simulink model "larix2"  (R2020b)
settings: Solver=FixedStepDiscrete  StartTime=0.0  StopTime=inf  FixedStep=0.002  RelTol=1e-3
PostLoadFcn:
  | load('ThrustTable.mat');
InitFcn:
  | run init.m
  | init()
values from neighbouring files (symbols this model uses):
  blimp = inertias()    [init.m]
  eul_0 = [-45*pi/180 0 0]    [init.m]
  g = 9.810    (= 9.81)    [init.m]
libraries: slpidlib x10, simulink x10, sharedtransform x1
settings Model: Creator=ac114611  LastModifiedBy=wendelin
settings DataIOCC: ReturnWorkspaceOutputs=off
settings OptimizationCC: BlockReduction=off  DefaultParameterBehavior=Inlined  BufferReuse=off  EnhancedBackFolding=on  PassReuseOutputArgsAs=Individual arguments  MaxStackSize=64  OptimizeBlockOrder=speed  DifferentSizesBufferReuse=on  EfficientTunableParamExpr=on
settings DebuggingCC: ParameterPrecisionLossMsg=none  ParameterTunabilityLossMsg=error  ArithmeticOperatorsInVariantConditions=warning
settings HardwareCC: ProdBitPerPointer=32  ProdBitPerSizeT=32  ProdBitPerPtrDiffT=32  ProdLargestAtomicInteger=Long  ProdLargestAtomicFloat=Double  ProdWordSize=32  ProdHWDeviceType=ARM Compatible->ARM Cortex  TargetBitPerLong=64  TargetBitPerPointer=64  TargetBitPerSizeT=64  TargetBitPerPtrDiffT=64  TargetLongLongMode=on  TargetIntDivRoundTo=Zero  TargetEndianess=LittleEndian  TargetWordSize=64  TargetHWDeviceType=MATLAB Host  ProdEqTarget=off
settings SFSimCC: SimUseLocalCustomCode=off  MATLABDynamicMemAlloc=off  CustomCodeUndefinedFunction=UseInterfaceOnly
settings RTWCC: Description=Embedded Coder  SystemTargetFile=ert.tlc  GenCodeOnly=on  PackageName=larix2_codegen.zip  TemplateMakefile=ert_default_tmf  RTWUseLocalCustomCode=off  Toolchain=GNU gcc/g++ | gmake (64-bit Linux)  IncludeHyperlinkInReport=on  GenerateCodeMetricsReport=on
settings CodeAppCC: ForceParamTrailComments=on  IgnoreCustomStorageClasses=off  OperatorAnnotations=on  SimulinkDataObjDesc=on  SFDataObjDesc=on  InsertBlockDesc=on
settings ERTTargetCC: TargetLangStandard=C99 (ISO)  SupportVariableSizeSignals=on  InlinedParameterPlacement=NonHierarchical  ERTCustomFileTemplate=example_file_process.tlc

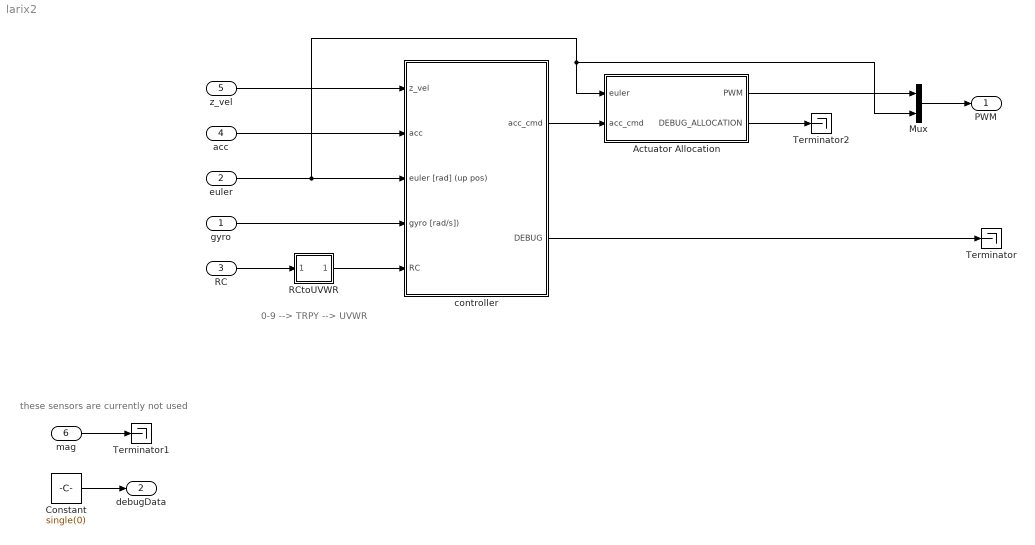
== system larix2 ==
  note: 0-9 --> TRPY --> UVWR
  note: these sensors are currently not used
  gyro : Inport  OutDataTypeStr=single  PortDimensions=3
  euler : Inport  Port=2  OutDataTypeStr=single  PortDimensions=3
  RC : Inport  Port=3  OutDataTypeStr=single  PortDimensions=10
  acc : Inport  Port=4  OutDataTypeStr=single  PortDimensions=3
  "z_vel " : Inport  Port=5  OutDataTypeStr=single  PortDimensions=1
  mag : Inport  Port=6  OutDataTypeStr=single  PortDimensions=3
  Actuator Allocation : Subsystem
  Constant : Constant  Value=single(0)
  Mux : Mux  Inputs=2
  RCtoUVWR : Subsystem
  Terminator : Terminator
  Terminator1 : Terminator
  Terminator2 : Terminator
  controller : Subsystem
  PWM : Outport  OutDataTypeStr=single  VectorParamsAs1DForOutWhenUnconnected=off
  debugData : Outport  Port=2
  wires:
  mag/1 -> Terminator1/1
  Actuator Allocation/1(PWM) -> Mux/1
  "z_vel "/1 -> controller/1(z_vel)
  acc/1 -> controller/2(acc)
  euler/1 -> Mux/2, Actuator Allocation/1(euler), controller/3(euler [rad] (up pos))
  gyro/1 -> controller/4(gyro [rad/s]))
  Constant/1 -> debugData/1
  Mux/1 -> PWM/1
  controller/2(DEBUG) -> Terminator/1
  controller/1(acc_cmd) -> Actuator Allocation/2(acc_cmd)
  RC/1 -> RCtoUVWR/1(RC)
  RCtoUVWR/1(Out1) -> controller/5(RC)
  Actuator Allocation/2(DEBUG_ALLOCATION) -> Terminator2/1

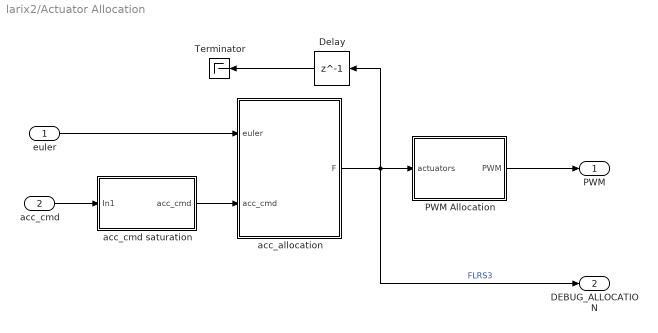
== system larix2/Actuator Allocation ==
  euler : Inport
  acc_cmd : Inport  Port=2
  Delay : Delay  DelayLength=1
  PWM Allocation : Subsystem
  Terminator : Terminator
  acc_allocation : MATLAB Function  TreatAsAtomicUnit=on
  acc_cmd saturation : Subsystem
  PWM : Outport
  DEBUG_ALLOCATION : Outport  Port=2
  wires:
  acc_cmd/1 -> acc_cmd saturation/1(In1)
  acc_cmd saturation/1(acc_cmd) -> acc_allocation/2(acc_cmd)
  euler/1 -> acc_allocation/1(euler)
  PWM Allocation/1(PWM) -> PWM/1
  acc_allocation/1(F) -> DEBUG_ALLOCATION/1, PWM Allocation/1(actuators), Delay/1  "FLRS3"
  Delay/1 -> Terminator/1

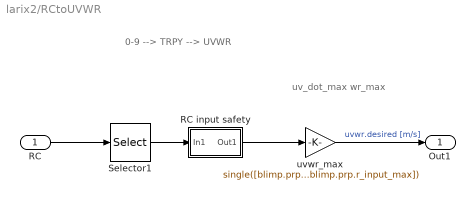
== system larix2/RCtoUVWR ==
  note: uv_dot_max
      | wr_max
  note: 0-9 --> TRPY --> UVWR
  RC : Inport  PortDimensions=10
  RC input safety : Subsystem
  Selector1 : Selector  IndexMode=Zero-based  InputPortWidth=10  IndexOptions=Index vector (dialog)  Indices=[2 1 0 3]  OutputSizes=1
  uvwr_max : Gain  Gain=single([blimp.prp.du_input_max, blimp.prp.dv_input_max, blimp.prp.w_input_max, blimp.prp.r_input_max])
  Out1 : Outport
  wires:
  RC/1 -> Selector1/1
  RC input safety/1(Out1) -> uvwr_max/1
  Selector1/1 -> RC input safety/1(In1)
  uvwr_max/1 -> Out1/1  "uvwr.desired [m/s]"

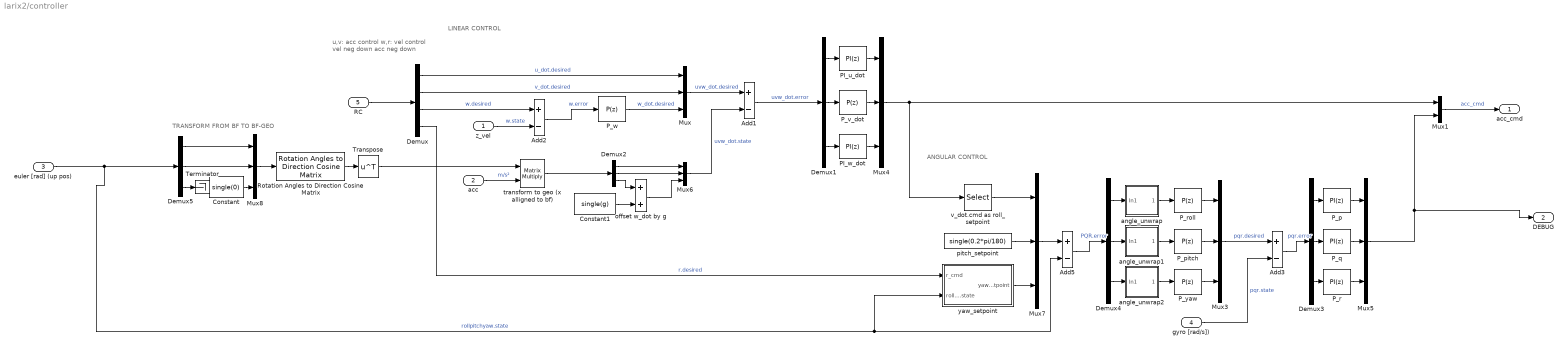
== system larix2/controller ==
  note: TRANSFORM FROM BF TO BF-GEO
  note: u,v: acc control
      | w,r: vel control
      |
      | vel neg down
      | acc neg down
  note: LINEAR CONTROL
  note: ANGULAR CONTROL
  z_vel : Inport  PortDimensions=1
  acc : Inport  Port=2  PortDimensions=3
  euler [rad] (up pos) : Inport  Port=3  PortDimensions=3
  gyro [rad/s]) : Inport  Port=4  PortDimensions=3
  RC : Inport  Port=5
  Add{1..3,5} (4 alike) : Sum  Inputs=+-
  Constant : Constant  Value=single(0)
  Constant1 : Constant  Value=single(g)
  Demux : Demux
  Demux{1..5} (5 alike) : Demux  Outputs=3
  Mux{,3..8} (7 alike) : Mux  Inputs=3
  Mux1 : Mux  Inputs=2
  PI_u_dot : slpidlib/PID Controller  Controller=PI  Form=Parallel  TimeDomain=Discrete-time  UseExternalTs=off  SampleTime=-1  IntegratorMethod=Trapezoidal  FilterMethod=Forward Euler  ControllerParametersSource=internal  P=0.15  I=0.05  D=0  UseFilter=on  N=100  TunerSelectOption=Transfer Function Based (PID Tuner App)  InitialConditionSource=internal  InitialConditionForIntegrator=0  InitialConditionForFilter=0  DifferentiatorICPrevScaledInput=0  ExternalReset=none  TrackingMode=off  Kt=1  LimitOutput=off  SatLimitsSource=internal  UpperSaturationLimit=0.4*g  LowerSaturationLimit=-0.4*g  LinearizeAsGain=off  AntiWindupMode=none  Kb=1  POutMin=[]  POutMax=[]  IOutMin=[]  IOutMax=[]  DOutMin=[]  DOutMax=[]  NOutMin=[]  NOutMax=[]  SumOutMin=[]  SumOutMax=[]  SaturationOutMin=[]  SaturationOutMax=[]  PParamMin=[]  PParamMax=[]  IParamMin=[]  IParamMax=[]  DParamMin=[]  DParamMax=[]  NParamMin=[]  NParamMax=[]  KbParamMin=[]  KbParamMax=[]  KtParamMin=[]  KtParamMax=[]  KbOutMin=[]  KbOutMax=[]  KtOutMin=[]  KtOutMax=[]  IntegratorOutMin=[]  IntegratorOutMax=[]  FilterOutMin=[]  FilterOutMax=[]  SumI1OutMin=[]  SumI1OutMax=[]  SumI2OutMin=[]  SumI2OutMax=[]  SumI3OutMin=[]  SumI3OutMax=[]  SumI4OutMin=[]  SumI4OutMax=[]  SumDOutMin=[]  SumDOutMax=[]  DifferentiatorOutMin=[]  DifferentiatorOutMax=[]  FilterDiffOutCoefMin=[]  FilterDiffOutCoefMax=[]  ReciprocalOutMin=[]  ReciprocalOutMax=[]  SumDenOutMin=[]  SumDenOutMax=[]  SumNumOutMin=[]  SumNumOutMax=[]  DivideOutMin=[]  DivideOutMax=[]  UdiffTsProdOutMin=[]  UdiffTsProdOutMax=[]  NTsProdOutMin=[]  NTsProdOutMax=[]  UintegralTsProdOutMin=[]  UintegralTsProdOutMax=[]  UngainTsProdOutMin=[]  UngainTsProdOutMax=[]  IntegratorContinuousStateAttributes=''  IntegratorStateMustResolveToSignalObject=off  IntegratorRTWStateStorageClass=Auto  FilterContinuousStateAttributes=''  FilterStateMustResolveToSignalObject=off  FilterRTWStateStorageClass=Auto  ParallelPVariant=InternalParameters  IdealPVariant=Disabled  IVariant=InternalParameters  DVariant=Disabled  IntegratorVariant=Discrete  SatVariant=Disabled  AWVariant=Passthrough  PCopyVariant=Disabled  TRVariant=Disabled  FdbkBlocksVariant=Forward  IdealPFdbkVariant=Disabled  SatFdbkVariant=Disabled  DerivativeFilterVariant=Disabled  NVariant=Disabled  NCopyVariant=Disabled_SignalSpec  FilterICVariant=Disabled  IntegratorICVariant=InternalICs  ExternalResetVariant=Disabled  TRSumVariant=Passthrough  SumFdbkVariant=Disabled  SumVariant=Sum_PI  TsampFilterVariant=InternalTs  TsampNgainVariant=Passthrough  TsampIntegralVariant=Passthrough  ExternalSaturationOutDataTypeStr=Inherit: Same as second input
  PI_w_dot : slpidlib/PID Controller  Controller=PI  Form=Parallel  TimeDomain=Discrete-time  UseExternalTs=off  SampleTime=-1  IntegratorMethod=Forward Euler  FilterMethod=Forward Euler  ControllerParametersSource=internal  P=1.8  I=1.4  D=0  UseFilter=on  N=100  TunerSelectOption=Transfer Function Based (PID Tuner App)  InitialConditionSource=internal  InitialConditionForIntegrator=0  InitialConditionForFilter=0  DifferentiatorICPrevScaledInput=0  ExternalReset=none  TrackingMode=off  Kt=1  LimitOutput=off  SatLimitsSource=internal  UpperSaturationLimit=inf  LowerSaturationLimit=0  LinearizeAsGain=off  AntiWindupMode=none  Kb=1  POutMin=[]  POutMax=[]  IOutMin=[]  IOutMax=[]  DOutMin=[]  DOutMax=[]  NOutMin=[]  NOutMax=[]  SumOutMin=[]  SumOutMax=[]  SaturationOutMin=[]  SaturationOutMax=[]  PParamMin=[]  PParamMax=[]  IParamMin=[]  IParamMax=[]  DParamMin=[]  DParamMax=[]  NParamMin=[]  NParamMax=[]  KbParamMin=[]  KbParamMax=[]  KtParamMin=[]  KtParamMax=[]  KbOutMin=[]  KbOutMax=[]  KtOutMin=[]  KtOutMax=[]  IntegratorOutMin=[]  IntegratorOutMax=[]  FilterOutMin=[]  FilterOutMax=[]  SumI1OutMin=[]  SumI1OutMax=[]  SumI2OutMin=[]  SumI2OutMax=[]  SumI3OutMin=[]  SumI3OutMax=[]  SumI4OutMin=[]  SumI4OutMax=[]  SumDOutMin=[]  SumDOutMax=[]  DifferentiatorOutMin=[]  DifferentiatorOutMax=[]  FilterDiffOutCoefMin=[]  FilterDiffOutCoefMax=[]  ReciprocalOutMin=[]  ReciprocalOutMax=[]  SumDenOutMin=[]  SumDenOutMax=[]  SumNumOutMin=[]  SumNumOutMax=[]  DivideOutMin=[]  DivideOutMax=[]  UdiffTsProdOutMin=[]  UdiffTsProdOutMax=[]  NTsProdOutMin=[]  NTsProdOutMax=[]  UintegralTsProdOutMin=[]  UintegralTsProdOutMax=[]  UngainTsProdOutMin=[]  UngainTsProdOutMax=[]  IntegratorContinuousStateAttributes=''  IntegratorStateMustResolveToSignalObject=off  IntegratorRTWStateStorageClass=Auto  FilterContinuousStateAttributes=''  FilterStateMustResolveToSignalObject=off  FilterRTWStateStorageClass=Auto  ParallelPVariant=InternalParameters  IdealPVariant=Disabled  IVariant=InternalParameters  DVariant=Disabled  IntegratorVariant=Discrete  SatVariant=Disabled  AWVariant=Passthrough  PCopyVariant=Disabled  TRVariant=Disabled  FdbkBlocksVariant=Forward  IdealPFdbkVariant=Disabled  SatFdbkVariant=Disabled  DerivativeFilterVariant=Disabled  NVariant=Disabled  NCopyVariant=Disabled_SignalSpec  FilterICVariant=Disabled  IntegratorICVariant=InternalICs  ExternalResetVariant=Disabled  TRSumVariant=Passthrough  SumFdbkVariant=Disabled  SumVariant=Sum_PI  TsampFilterVariant=InternalTs  TsampNgainVariant=Passthrough  TsampIntegralVariant=Passthrough  ExternalSaturationOutDataTypeStr=Inherit: Same as second input
  P_p : slpidlib/PID Controller  Controller=PI  Form=Parallel  TimeDomain=Discrete-time  UseExternalTs=off  SampleTime=-1  IntegratorMethod=Forward Euler  FilterMethod=Forward Euler  ControllerParametersSource=internal  P=0.4  I=10  D=0  UseFilter=on  N=100  TunerSelectOption=Transfer Function Based (PID Tuner App)  InitialConditionSource=internal  InitialConditionForIntegrator=0  InitialConditionForFilter=0  DifferentiatorICPrevScaledInput=0  ExternalReset=none  TrackingMode=off  Kt=1  LimitOutput=off  SatLimitsSource=internal  UpperSaturationLimit=inf  LowerSaturationLimit=-inf  LinearizeAsGain=on  AntiWindupMode=none  Kb=1  POutMin=[]  POutMax=[]  IOutMin=[]  IOutMax=[]  DOutMin=[]  DOutMax=[]  NOutMin=[]  NOutMax=[]  SumOutMin=[]  SumOutMax=[]  SaturationOutMin=[]  SaturationOutMax=[]  PParamMin=[]  PParamMax=[]  IParamMin=[]  IParamMax=[]  DParamMin=[]  DParamMax=[]  NParamMin=[]  NParamMax=[]  KbParamMin=[]  KbParamMax=[]  KtParamMin=[]  KtParamMax=[]  KbOutMin=[]  KbOutMax=[]  KtOutMin=[]  KtOutMax=[]  IntegratorOutMin=[]  IntegratorOutMax=[]  FilterOutMin=[]  FilterOutMax=[]  SumI1OutMin=[]  SumI1OutMax=[]  SumI2OutMin=[]  SumI2OutMax=[]  SumI3OutMin=[]  SumI3OutMax=[]  SumI4OutMin=[]  SumI4OutMax=[]  SumDOutMin=[]  SumDOutMax=[]  DifferentiatorOutMin=[]  DifferentiatorOutMax=[]  FilterDiffOutCoefMin=[]  FilterDiffOutCoefMax=[]  ReciprocalOutMin=[]  ReciprocalOutMax=[]  SumDenOutMin=[]  SumDenOutMax=[]  SumNumOutMin=[]  SumNumOutMax=[]  DivideOutMin=[]  DivideOutMax=[]  UdiffTsProdOutMin=[]  UdiffTsProdOutMax=[]  NTsProdOutMin=[]  NTsProdOutMax=[]  UintegralTsProdOutMin=[]  UintegralTsProdOutMax=[]  UngainTsProdOutMin=[]  UngainTsProdOutMax=[]  IntegratorContinuousStateAttributes=''  IntegratorStateMustResolveToSignalObject=off  IntegratorRTWStateStorageClass=Auto  FilterContinuousStateAttributes=''  FilterStateMustResolveToSignalObject=off  FilterRTWStateStorageClass=Auto  ParallelPVariant=InternalParameters  IdealPVariant=Disabled  IVariant=InternalParameters  DVariant=Disabled  IntegratorVariant=Discrete  SatVariant=Disabled  AWVariant=Passthrough  PCopyVariant=Disabled  TRVariant=Disabled  FdbkBlocksVariant=Forward  IdealPFdbkVariant=Disabled  SatFdbkVariant=Disabled  DerivativeFilterVariant=Disabled  NVariant=Disabled  NCopyVariant=Disabled_SignalSpec  FilterICVariant=Disabled  IntegratorICVariant=InternalICs  ExternalResetVariant=Disabled  TRSumVariant=Passthrough  SumFdbkVariant=Disabled  SumVariant=Sum_PI  TsampFilterVariant=InternalTs  TsampNgainVariant=Passthrough  TsampIntegralVariant=Passthrough  ExternalSaturationOutDataTypeStr=Inherit: Same as second input
  P_pitch : slpidlib/PID Controller  Controller=P  Form=Parallel  TimeDomain=Discrete-time  UseExternalTs=off  SampleTime=-1  IntegratorMethod=Forward Euler  FilterMethod=Forward Euler  ControllerParametersSource=internal  P=1  I=0  D=0  UseFilter=on  N=100  TunerSelectOption=Transfer Function Based (PID Tuner App)  InitialConditionSource=internal  InitialConditionForIntegrator=0  InitialConditionForFilter=0  DifferentiatorICPrevScaledInput=0  ExternalReset=none  TrackingMode=off  Kt=1  LimitOutput=off  SatLimitsSource=internal  UpperSaturationLimit=inf  LowerSaturationLimit=-inf  LinearizeAsGain=on  AntiWindupMode=none  Kb=1  POutMin=[]  POutMax=[]  IOutMin=[]  IOutMax=[]  DOutMin=[]  DOutMax=[]  NOutMin=[]  NOutMax=[]  SumOutMin=[]  SumOutMax=[]  SaturationOutMin=[]  SaturationOutMax=[]  PParamMin=[]  PParamMax=[]  IParamMin=[]  IParamMax=[]  DParamMin=[]  DParamMax=[]  NParamMin=[]  NParamMax=[]  KbParamMin=[]  KbParamMax=[]  KtParamMin=[]  KtParamMax=[]  KbOutMin=[]  KbOutMax=[]  KtOutMin=[]  KtOutMax=[]  IntegratorOutMin=[]  IntegratorOutMax=[]  FilterOutMin=[]  FilterOutMax=[]  SumI1OutMin=[]  SumI1OutMax=[]  SumI2OutMin=[]  SumI2OutMax=[]  SumI3OutMin=[]  SumI3OutMax=[]  SumI4OutMin=[]  SumI4OutMax=[]  SumDOutMin=[]  SumDOutMax=[]  DifferentiatorOutMin=[]  DifferentiatorOutMax=[]  FilterDiffOutCoefMin=[]  FilterDiffOutCoefMax=[]  ReciprocalOutMin=[]  ReciprocalOutMax=[]  SumDenOutMin=[]  SumDenOutMax=[]  SumNumOutMin=[]  SumNumOutMax=[]  DivideOutMin=[]  DivideOutMax=[]  UdiffTsProdOutMin=[]  UdiffTsProdOutMax=[]  NTsProdOutMin=[]  NTsProdOutMax=[]  UintegralTsProdOutMin=[]  UintegralTsProdOutMax=[]  UngainTsProdOutMin=[]  UngainTsProdOutMax=[]  IntegratorContinuousStateAttributes=''  IntegratorStateMustResolveToSignalObject=off  IntegratorRTWStateStorageClass=Auto  FilterContinuousStateAttributes=''  FilterStateMustResolveToSignalObject=off  FilterRTWStateStorageClass=Auto  ParallelPVariant=InternalParameters  IdealPVariant=Disabled  IVariant=Disabled  DVariant=Disabled  IntegratorVariant=Disabled  SatVariant=Disabled  AWVariant=Disabled  PCopyVariant=Disabled  TRVariant=Disabled  FdbkBlocksVariant=Forward  IdealPFdbkVariant=Disabled  SatFdbkVariant=Disabled  DerivativeFilterVariant=Disabled  NVariant=Disabled  NCopyVariant=Disabled_SignalSpec  FilterICVariant=Disabled  IntegratorICVariant=Disabled  ExternalResetVariant=Disabled  TRSumVariant=Passthrough  SumFdbkVariant=Disabled  SumVariant=Passthrough_P  TsampFilterVariant=InternalTs  TsampNgainVariant=Passthrough  TsampIntegralVariant=Disabled_SignalSpec  ExternalSaturationOutDataTypeStr=Inherit: Same as second input
  P_q : slpidlib/PID Controller  Controller=PI  Form=Parallel  TimeDomain=Discrete-time  UseExternalTs=off  SampleTime=-1  IntegratorMethod=Forward Euler  FilterMethod=Forward Euler  ControllerParametersSource=internal  P=1  I=0  D=0  UseFilter=on  N=100  TunerSelectOption=Transfer Function Based (PID Tuner App)  InitialConditionSource=internal  InitialConditionForIntegrator=0  InitialConditionForFilter=0  DifferentiatorICPrevScaledInput=0  ExternalReset=none  TrackingMode=off  Kt=1  LimitOutput=off  SatLimitsSource=internal  UpperSaturationLimit=inf  LowerSaturationLimit=-inf  LinearizeAsGain=on  AntiWindupMode=none  Kb=1  POutMin=[]  POutMax=[]  IOutMin=[]  IOutMax=[]  DOutMin=[]  DOutMax=[]  NOutMin=[]  NOutMax=[]  SumOutMin=[]  SumOutMax=[]  SaturationOutMin=[]  SaturationOutMax=[]  PParamMin=[]  PParamMax=[]  IParamMin=[]  IParamMax=[]  DParamMin=[]  DParamMax=[]  NParamMin=[]  NParamMax=[]  KbParamMin=[]  KbParamMax=[]  KtParamMin=[]  KtParamMax=[]  KbOutMin=[]  KbOutMax=[]  KtOutMin=[]  KtOutMax=[]  IntegratorOutMin=[]  IntegratorOutMax=[]  FilterOutMin=[]  FilterOutMax=[]  SumI1OutMin=[]  SumI1OutMax=[]  SumI2OutMin=[]  SumI2OutMax=[]  SumI3OutMin=[]  SumI3OutMax=[]  SumI4OutMin=[]  SumI4OutMax=[]  SumDOutMin=[]  SumDOutMax=[]  DifferentiatorOutMin=[]  DifferentiatorOutMax=[]  FilterDiffOutCoefMin=[]  FilterDiffOutCoefMax=[]  ReciprocalOutMin=[]  ReciprocalOutMax=[]  SumDenOutMin=[]  SumDenOutMax=[]  SumNumOutMin=[]  SumNumOutMax=[]  DivideOutMin=[]  DivideOutMax=[]  UdiffTsProdOutMin=[]  UdiffTsProdOutMax=[]  NTsProdOutMin=[]  NTsProdOutMax=[]  UintegralTsProdOutMin=[]  UintegralTsProdOutMax=[]  UngainTsProdOutMin=[]  UngainTsProdOutMax=[]  IntegratorContinuousStateAttributes=''  IntegratorStateMustResolveToSignalObject=off  IntegratorRTWStateStorageClass=Auto  FilterContinuousStateAttributes=''  FilterStateMustResolveToSignalObject=off  FilterRTWStateStorageClass=Auto  ParallelPVariant=InternalParameters  IdealPVariant=Disabled  IVariant=InternalParameters  DVariant=Disabled  IntegratorVariant=Discrete  SatVariant=Disabled  AWVariant=Passthrough  PCopyVariant=Disabled  TRVariant=Disabled  FdbkBlocksVariant=Forward  IdealPFdbkVariant=Disabled  SatFdbkVariant=Disabled  DerivativeFilterVariant=Disabled  NVariant=Disabled  NCopyVariant=Disabled_SignalSpec  FilterICVariant=Disabled  IntegratorICVariant=InternalICs  ExternalResetVariant=Disabled  TRSumVariant=Passthrough  SumFdbkVariant=Disabled  SumVariant=Sum_PI  TsampFilterVariant=InternalTs  TsampNgainVariant=Passthrough  TsampIntegralVariant=Passthrough  ExternalSaturationOutDataTypeStr=Inherit: Same as second input
  P_r : slpidlib/PID Controller  Controller=PI  Form=Parallel  TimeDomain=Discrete-time  UseExternalTs=off  SampleTime=-1  IntegratorMethod=Forward Euler  FilterMethod=Forward Euler  ControllerParametersSource=internal  P=0.5  I=0.2  D=0  UseFilter=on  N=100  TunerSelectOption=Transfer Function Based (PID Tuner App)  InitialConditionSource=internal  InitialConditionForIntegrator=0  InitialConditionForFilter=0  DifferentiatorICPrevScaledInput=0  ExternalReset=none  TrackingMode=off  Kt=1  LimitOutput=off  SatLimitsSource=internal  UpperSaturationLimit=inf  LowerSaturationLimit=-inf  LinearizeAsGain=on  AntiWindupMode=none  Kb=1  POutMin=[]  POutMax=[]  IOutMin=[]  IOutMax=[]  DOutMin=[]  DOutMax=[]  NOutMin=[]  NOutMax=[]  SumOutMin=[]  SumOutMax=[]  SaturationOutMin=[]  SaturationOutMax=[]  PParamMin=[]  PParamMax=[]  IParamMin=[]  IParamMax=[]  DParamMin=[]  DParamMax=[]  NParamMin=[]  NParamMax=[]  KbParamMin=[]  KbParamMax=[]  KtParamMin=[]  KtParamMax=[]  KbOutMin=[]  KbOutMax=[]  KtOutMin=[]  KtOutMax=[]  IntegratorOutMin=[]  IntegratorOutMax=[]  FilterOutMin=[]  FilterOutMax=[]  SumI1OutMin=[]  SumI1OutMax=[]  SumI2OutMin=[]  SumI2OutMax=[]  SumI3OutMin=[]  SumI3OutMax=[]  SumI4OutMin=[]  SumI4OutMax=[]  SumDOutMin=[]  SumDOutMax=[]  DifferentiatorOutMin=[]  DifferentiatorOutMax=[]  FilterDiffOutCoefMin=[]  FilterDiffOutCoefMax=[]  ReciprocalOutMin=[]  ReciprocalOutMax=[]  SumDenOutMin=[]  SumDenOutMax=[]  SumNumOutMin=[]  SumNumOutMax=[]  DivideOutMin=[]  DivideOutMax=[]  UdiffTsProdOutMin=[]  UdiffTsProdOutMax=[]  NTsProdOutMin=[]  NTsProdOutMax=[]  UintegralTsProdOutMin=[]  UintegralTsProdOutMax=[]  UngainTsProdOutMin=[]  UngainTsProdOutMax=[]  IntegratorContinuousStateAttributes=''  IntegratorStateMustResolveToSignalObject=off  IntegratorRTWStateStorageClass=Auto  FilterContinuousStateAttributes=''  FilterStateMustResolveToSignalObject=off  FilterRTWStateStorageClass=Auto  ParallelPVariant=InternalParameters  IdealPVariant=Disabled  IVariant=InternalParameters  DVariant=Disabled  IntegratorVariant=Discrete  SatVariant=Disabled  AWVariant=Passthrough  PCopyVariant=Disabled  TRVariant=Disabled  FdbkBlocksVariant=Forward  IdealPFdbkVariant=Disabled  SatFdbkVariant=Disabled  DerivativeFilterVariant=Disabled  NVariant=Disabled  NCopyVariant=Disabled_SignalSpec  FilterICVariant=Disabled  IntegratorICVariant=InternalICs  ExternalResetVariant=Disabled  TRSumVariant=Passthrough  SumFdbkVariant=Disabled  SumVariant=Sum_PI  TsampFilterVariant=InternalTs  TsampNgainVariant=Passthrough  TsampIntegralVariant=Passthrough  ExternalSaturationOutDataTypeStr=Inherit: Same as second input
  P_roll : slpidlib/PID Controller  Controller=P  Form=Parallel  TimeDomain=Discrete-time  UseExternalTs=off  SampleTime=-1  IntegratorMethod=Forward Euler  FilterMethod=Forward Euler  ControllerParametersSource=internal  P=2  I=0  D=0  UseFilter=on  N=100  TunerSelectOption=Transfer Function Based (PID Tuner App)  InitialConditionSource=internal  InitialConditionForIntegrator=0  InitialConditionForFilter=0  DifferentiatorICPrevScaledInput=0  ExternalReset=none  TrackingMode=off  Kt=1  LimitOutput=off  SatLimitsSource=internal  UpperSaturationLimit=inf  LowerSaturationLimit=-inf  LinearizeAsGain=on  AntiWindupMode=none  Kb=1  POutMin=[]  POutMax=[]  IOutMin=[]  IOutMax=[]  DOutMin=[]  DOutMax=[]  NOutMin=[]  NOutMax=[]  SumOutMin=[]  SumOutMax=[]  SaturationOutMin=[]  SaturationOutMax=[]  PParamMin=[]  PParamMax=[]  IParamMin=[]  IParamMax=[]  DParamMin=[]  DParamMax=[]  NParamMin=[]  NParamMax=[]  KbParamMin=[]  KbParamMax=[]  KtParamMin=[]  KtParamMax=[]  KbOutMin=[]  KbOutMax=[]  KtOutMin=[]  KtOutMax=[]  IntegratorOutMin=[]  IntegratorOutMax=[]  FilterOutMin=[]  FilterOutMax=[]  SumI1OutMin=[]  SumI1OutMax=[]  SumI2OutMin=[]  SumI2OutMax=[]  SumI3OutMin=[]  SumI3OutMax=[]  SumI4OutMin=[]  SumI4OutMax=[]  SumDOutMin=[]  SumDOutMax=[]  DifferentiatorOutMin=[]  DifferentiatorOutMax=[]  FilterDiffOutCoefMin=[]  FilterDiffOutCoefMax=[]  ReciprocalOutMin=[]  ReciprocalOutMax=[]  SumDenOutMin=[]  SumDenOutMax=[]  SumNumOutMin=[]  SumNumOutMax=[]  DivideOutMin=[]  DivideOutMax=[]  UdiffTsProdOutMin=[]  UdiffTsProdOutMax=[]  NTsProdOutMin=[]  NTsProdOutMax=[]  UintegralTsProdOutMin=[]  UintegralTsProdOutMax=[]  UngainTsProdOutMin=[]  UngainTsProdOutMax=[]  IntegratorContinuousStateAttributes=''  IntegratorStateMustResolveToSignalObject=off  IntegratorRTWStateStorageClass=Auto  FilterContinuousStateAttributes=''  FilterStateMustResolveToSignalObject=off  FilterRTWStateStorageClass=Auto  ParallelPVariant=InternalParameters  IdealPVariant=Disabled  IVariant=Disabled  DVariant=Disabled  IntegratorVariant=Disabled  SatVariant=Disabled  AWVariant=Disabled  PCopyVariant=Disabled  TRVariant=Disabled  FdbkBlocksVariant=Forward  IdealPFdbkVariant=Disabled  SatFdbkVariant=Disabled  DerivativeFilterVariant=Disabled  NVariant=Disabled  NCopyVariant=Disabled_SignalSpec  FilterICVariant=Disabled  IntegratorICVariant=Disabled  ExternalResetVariant=Disabled  TRSumVariant=Passthrough  SumFdbkVariant=Disabled  SumVariant=Passthrough_P  TsampFilterVariant=InternalTs  TsampNgainVariant=Passthrough  TsampIntegralVariant=Disabled_SignalSpec  ExternalSaturationOutDataTypeStr=Inherit: Same as second input
  P_v_dot : slpidlib/PID Controller  Controller=P  Form=Parallel  TimeDomain=Discrete-time  UseExternalTs=off  SampleTime=-1  IntegratorMethod=Forward Euler  FilterMethod=Forward Euler  ControllerParametersSource=internal  P=2.5 *pi/180  I=1  D=0  UseFilter=on  N=100  TunerSelectOption=Transfer Function Based (PID Tuner App)  InitialConditionSource=internal  InitialConditionForIntegrator=0  InitialConditionForFilter=0  DifferentiatorICPrevScaledInput=0  ExternalReset=none  TrackingMode=off  Kt=1  LimitOutput=off  SatLimitsSource=internal  UpperSaturationLimit=inf  LowerSaturationLimit=-inf  LinearizeAsGain=on  AntiWindupMode=none  Kb=1  POutMin=[]  POutMax=[]  IOutMin=[]  IOutMax=[]  DOutMin=[]  DOutMax=[]  NOutMin=[]  NOutMax=[]  SumOutMin=[]  SumOutMax=[]  SaturationOutMin=[]  SaturationOutMax=[]  PParamMin=[]  PParamMax=[]  IParamMin=[]  IParamMax=[]  DParamMin=[]  DParamMax=[]  NParamMin=[]  NParamMax=[]  KbParamMin=[]  KbParamMax=[]  KtParamMin=[]  KtParamMax=[]  KbOutMin=[]  KbOutMax=[]  KtOutMin=[]  KtOutMax=[]  IntegratorOutMin=[]  IntegratorOutMax=[]  FilterOutMin=[]  FilterOutMax=[]  SumI1OutMin=[]  SumI1OutMax=[]  SumI2OutMin=[]  SumI2OutMax=[]  SumI3OutMin=[]  SumI3OutMax=[]  SumI4OutMin=[]  SumI4OutMax=[]  SumDOutMin=[]  SumDOutMax=[]  DifferentiatorOutMin=[]  DifferentiatorOutMax=[]  FilterDiffOutCoefMin=[]  FilterDiffOutCoefMax=[]  ReciprocalOutMin=[]  ReciprocalOutMax=[]  SumDenOutMin=[]  SumDenOutMax=[]  SumNumOutMin=[]  SumNumOutMax=[]  DivideOutMin=[]  DivideOutMax=[]  UdiffTsProdOutMin=[]  UdiffTsProdOutMax=[]  NTsProdOutMin=[]  NTsProdOutMax=[]  UintegralTsProdOutMin=[]  UintegralTsProdOutMax=[]  UngainTsProdOutMin=[]  UngainTsProdOutMax=[]  IntegratorContinuousStateAttributes=''  IntegratorStateMustResolveToSignalObject=off  IntegratorRTWStateStorageClass=Auto  FilterContinuousStateAttributes=''  FilterStateMustResolveToSignalObject=off  FilterRTWStateStorageClass=Auto  ParallelPVariant=InternalParameters  IdealPVariant=Disabled  IVariant=Disabled  DVariant=Disabled  IntegratorVariant=Disabled  SatVariant=Disabled  AWVariant=Disabled  PCopyVariant=Disabled  TRVariant=Disabled  FdbkBlocksVariant=Forward  IdealPFdbkVariant=Disabled  SatFdbkVariant=Disabled  DerivativeFilterVariant=Disabled  NVariant=Disabled  NCopyVariant=Disabled_SignalSpec  FilterICVariant=Disabled  IntegratorICVariant=Disabled  ExternalResetVariant=Disabled  TRSumVariant=Passthrough  SumFdbkVariant=Disabled  SumVariant=Passthrough_P  TsampFilterVariant=InternalTs  TsampNgainVariant=Passthrough  TsampIntegralVariant=Disabled_SignalSpec  ExternalSaturationOutDataTypeStr=Inherit: Same as second input
  P_w : slpidlib/PID Controller  Controller=P  Form=Parallel  TimeDomain=Discrete-time  UseExternalTs=off  SampleTime=-1  IntegratorMethod=Forward Euler  FilterMethod=Forward Euler  ControllerParametersSource=internal  P=1.3  I=0  D=0  UseFilter=on  N=100  TunerSelectOption=Transfer Function Based (PID Tuner App)  InitialConditionSource=internal  InitialConditionForIntegrator=0  InitialConditionForFilter=0  DifferentiatorICPrevScaledInput=0  ExternalReset=none  TrackingMode=off  Kt=1  LimitOutput=off  SatLimitsSource=internal  UpperSaturationLimit=inf  LowerSaturationLimit=-inf  LinearizeAsGain=off  AntiWindupMode=none  Kb=1  POutMin=[]  POutMax=[]  IOutMin=[]  IOutMax=[]  DOutMin=[]  DOutMax=[]  NOutMin=[]  NOutMax=[]  SumOutMin=[]  SumOutMax=[]  SaturationOutMin=[]  SaturationOutMax=[]  PParamMin=[]  PParamMax=[]  IParamMin=[]  IParamMax=[]  DParamMin=[]  DParamMax=[]  NParamMin=[]  NParamMax=[]  KbParamMin=[]  KbParamMax=[]  KtParamMin=[]  KtParamMax=[]  KbOutMin=[]  KbOutMax=[]  KtOutMin=[]  KtOutMax=[]  IntegratorOutMin=[]  IntegratorOutMax=[]  FilterOutMin=[]  FilterOutMax=[]  SumI1OutMin=[]  SumI1OutMax=[]  SumI2OutMin=[]  SumI2OutMax=[]  SumI3OutMin=[]  SumI3OutMax=[]  SumI4OutMin=[]  SumI4OutMax=[]  SumDOutMin=[]  SumDOutMax=[]  DifferentiatorOutMin=[]  DifferentiatorOutMax=[]  FilterDiffOutCoefMin=[]  FilterDiffOutCoefMax=[]  ReciprocalOutMin=[]  ReciprocalOutMax=[]  SumDenOutMin=[]  SumDenOutMax=[]  SumNumOutMin=[]  SumNumOutMax=[]  DivideOutMin=[]  DivideOutMax=[]  UdiffTsProdOutMin=[]  UdiffTsProdOutMax=[]  NTsProdOutMin=[]  NTsProdOutMax=[]  UintegralTsProdOutMin=[]  UintegralTsProdOutMax=[]  UngainTsProdOutMin=[]  UngainTsProdOutMax=[]  IntegratorContinuousStateAttributes=''  IntegratorStateMustResolveToSignalObject=off  IntegratorRTWStateStorageClass=Auto  FilterContinuousStateAttributes=''  FilterStateMustResolveToSignalObject=off  FilterRTWStateStorageClass=Auto  ParallelPVariant=InternalParameters  IdealPVariant=Disabled  IVariant=Disabled  DVariant=Disabled  IntegratorVariant=Disabled  SatVariant=Disabled  AWVariant=Disabled  PCopyVariant=Disabled  TRVariant=Disabled  FdbkBlocksVariant=Forward  IdealPFdbkVariant=Disabled  SatFdbkVariant=Disabled  DerivativeFilterVariant=Disabled  NVariant=Disabled  NCopyVariant=Disabled_SignalSpec  FilterICVariant=Disabled  IntegratorICVariant=Disabled  ExternalResetVariant=Disabled  TRSumVariant=Passthrough  SumFdbkVariant=Disabled  SumVariant=Passthrough_P  TsampFilterVariant=InternalTs  TsampNgainVariant=Passthrough  TsampIntegralVariant=Disabled_SignalSpec  ExternalSaturationOutDataTypeStr=Inherit: Same as second input
  P_yaw : slpidlib/PID Controller  Controller=P  Form=Parallel  TimeDomain=Discrete-time  UseExternalTs=off  SampleTime=-1  IntegratorMethod=Forward Euler  FilterMethod=Forward Euler  ControllerParametersSource=internal  P=1.7  I=0  D=0  UseFilter=on  N=100  TunerSelectOption=Transfer Function Based (PID Tuner App)  InitialConditionSource=internal  InitialConditionForIntegrator=0  InitialConditionForFilter=0  DifferentiatorICPrevScaledInput=0  ExternalReset=none  TrackingMode=off  Kt=1  LimitOutput=off  SatLimitsSource=internal  UpperSaturationLimit=inf  LowerSaturationLimit=-inf  LinearizeAsGain=on  AntiWindupMode=none  Kb=1  POutMin=[]  POutMax=[]  IOutMin=[]  IOutMax=[]  DOutMin=[]  DOutMax=[]  NOutMin=[]  NOutMax=[]  SumOutMin=[]  SumOutMax=[]  SaturationOutMin=[]  SaturationOutMax=[]  PParamMin=[]  PParamMax=[]  IParamMin=[]  IParamMax=[]  DParamMin=[]  DParamMax=[]  NParamMin=[]  NParamMax=[]  KbParamMin=[]  KbParamMax=[]  KtParamMin=[]  KtParamMax=[]  KbOutMin=[]  KbOutMax=[]  KtOutMin=[]  KtOutMax=[]  IntegratorOutMin=[]  IntegratorOutMax=[]  FilterOutMin=[]  FilterOutMax=[]  SumI1OutMin=[]  SumI1OutMax=[]  SumI2OutMin=[]  SumI2OutMax=[]  SumI3OutMin=[]  SumI3OutMax=[]  SumI4OutMin=[]  SumI4OutMax=[]  SumDOutMin=[]  SumDOutMax=[]  DifferentiatorOutMin=[]  DifferentiatorOutMax=[]  FilterDiffOutCoefMin=[]  FilterDiffOutCoefMax=[]  ReciprocalOutMin=[]  ReciprocalOutMax=[]  SumDenOutMin=[]  SumDenOutMax=[]  SumNumOutMin=[]  SumNumOutMax=[]  DivideOutMin=[]  DivideOutMax=[]  UdiffTsProdOutMin=[]  UdiffTsProdOutMax=[]  NTsProdOutMin=[]  NTsProdOutMax=[]  UintegralTsProdOutMin=[]  UintegralTsProdOutMax=[]  UngainTsProdOutMin=[]  UngainTsProdOutMax=[]  IntegratorContinuousStateAttributes=''  IntegratorStateMustResolveToSignalObject=off  IntegratorRTWStateStorageClass=Auto  FilterContinuousStateAttributes=''  FilterStateMustResolveToSignalObject=off  FilterRTWStateStorageClass=Auto  ParallelPVariant=InternalParameters  IdealPVariant=Disabled  IVariant=Disabled  DVariant=Disabled  IntegratorVariant=Disabled  SatVariant=Disabled  AWVariant=Disabled  PCopyVariant=Disabled  TRVariant=Disabled  FdbkBlocksVariant=Forward  IdealPFdbkVariant=Disabled  SatFdbkVariant=Disabled  DerivativeFilterVariant=Disabled  NVariant=Disabled  NCopyVariant=Disabled_SignalSpec  FilterICVariant=Disabled  IntegratorICVariant=Disabled  ExternalResetVariant=Disabled  TRSumVariant=Passthrough  SumFdbkVariant=Disabled  SumVariant=Passthrough_P  TsampFilterVariant=InternalTs  TsampNgainVariant=Passthrough  TsampIntegralVariant=Disabled_SignalSpec  ExternalSaturationOutDataTypeStr=Inherit: Same as second input
  Rotation Angles to Direction Cosine Matrix : sharedtransform/Rotation Angles to Direction Cosine Matrix  rotationOrder=XYZ  aMode=aMode
      settings: SourceProductBaseCode=AE,PW,MT,UV,VE,VP
  Terminator : Terminator
  Transpose : Math  Operator=transpose  SaturateOnIntegerOverflow=on
  angle_unwrap : Subsystem
  angle_unwrap1 : Subsystem
  angle_unwrap2 : Subsystem
  offset w_dot by g : Sum
  pitch_setpoint : Constant  Value=single(0.2*pi/180)
  transform to geo (x alligned to bf) : Product  Multiplication=Matrix(*)
  v_dot.cmd as roll_setpoint : Selector  InputPortWidth=3  IndexOptions=Index vector (dialog)  Indices=[2]  OutputSizes=1
  yaw_setpoint : Subsystem
  acc_cmd : Outport
  DEBUG : Outport  Port=2
  wires:
  Mux1/1 -> acc_cmd/1  "acc_cmd"
  P_r/1 -> Mux5/3
  Mux6/1 -> Add1/2  "uvw_dot.state"
  Demux/1 -> Mux/1  "u_dot.desired"
  offset w_dot by g/1 -> Mux6/3
  Add3/1 -> Demux3/1  "pqr.error"
  Demux2/3 -> offset w_dot by g/1
  Add2/1 -> P_w/1  "w.error"
  Demux3/2 -> P_q/1
  P_p/1 -> Mux5/1
  Demux/4 -> yaw_setpoint/1(r_cmd)  "r.desired"
  Demux1/3 -> PI_w_dot/1
  Constant1/1 -> offset w_dot by g/2
  Demux/2 -> Mux/2  "v_dot.desired"
  P_w/1 -> Mux/3  "w_dot.desired"
  Mux4/1 -> Mux1/1, v_dot.cmd as roll_setpoint/1
  Demux3/3 -> P_r/1
  z_vel/1 -> Add2/2  "w.state"
  Demux3/1 -> P_p/1
  PI_w_dot/1 -> Mux4/3
  P_q/1 -> Mux5/2
  gyro [rad/s])/1 -> Add3/2  "pqr.state"
  euler [rad] (up pos)/1 -> Demux5/1, yaw_setpoint/2(rollpitchyaw.state), Add5/2  "rollpitchyaw.state"
  PI_u_dot/1 -> Mux4/1
  Demux1/2 -> P_v_dot/1
  Mux/1 -> Add1/1  "uvw_dot.desired"
  RC/1 -> Demux/1
  Add5/1 -> Demux4/1  "PQR.error"
  Add1/1 -> Demux1/1  "uvw_dot.error"
  acc/1 -> transform to geo (x alligned to bf)/2  "m/s²"
  Demux/3 -> Add2/1  "w.desired"
  P_roll/1 -> Mux3/1
  Demux1/1 -> PI_u_dot/1
  Mux3/1 -> Add3/1  "pqr.desired"
  P_pitch/1 -> Mux3/2
  pitch_setpoint/1 -> Mux7/2
  Mux7/1 -> Add5/1
  v_dot.cmd as roll_setpoint/1 -> Mux7/1
  Rotation Angles to Direction Cosine Matrix/1 -> Transpose/1
  Demux5/1 -> Mux8/1
  Demux5/2 -> Mux8/2
  Demux5/3 -> Terminator/1
  Constant/1 -> Mux8/3
  Mux8/1 -> Rotation Angles to Direction Cosine Matrix/1
  Demux2/1 -> Mux6/1
  transform to geo (x alligned to bf)/1 -> Demux2/1
  Demux2/2 -> Mux6/2
  yaw_setpoint/1(yaw_setpoint) -> Mux7/3
  P_yaw/1 -> Mux3/3
  Demux4/3 -> angle_unwrap2/1(In1)
  P_v_dot/1 -> Mux4/2
  Transpose/1 -> transform to geo (x alligned to bf)/1
  Demux4/2 -> angle_unwrap1/1(In1)
  Demux4/1 -> angle_unwrap/1(In1)
  angle_unwrap/1(Out1) -> P_roll/1
  angle_unwrap1/1(Out1) -> P_pitch/1
  angle_unwrap2/1(Out1) -> P_yaw/1
  Mux5/1 -> DEBUG/1, Mux1/2

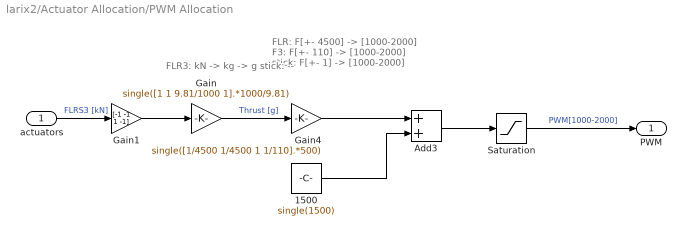
== system larix2/Actuator Allocation/PWM Allocation ==
  note: FLR: F[+- 4500] -> [1000-2000]
      | F3:    F[+- 110]   -> [1000-2000]
      | stick: F[+- 1]       -> [1000-2000]
  note: FLR3: kN -> kg -> g
      | stick: --
  actuators : Inport
  1500 : Constant  Value=single(1500)
  Add3 : Sum
  Gain : Gain  Gain=single([1 1 9.81/1000 1].*1000/9.81)
  Gain1 : Gain  Gain=[-1 -1 1 -1]
  Gain4 : Gain  Gain=single([1/4500 1/4500 1 1/110].*500)
  Saturation : Saturate  UpperLimit=2000  LowerLimit=1000
  PWM : Outport  VectorParamsAs1DForOutWhenUnconnected=off
  wires:
  actuators/1 -> Gain1/1  "FLRS3 [kN]"
  Saturation/1 -> PWM/1  "PWM[1000-2000]"
  Gain/1 -> Gain4/1  "Thrust [g]"
  Gain4/1 -> Add3/1
  1500/1 -> Add3/2
  Add3/1 -> Saturation/1
  Gain1/1 -> Gain/1

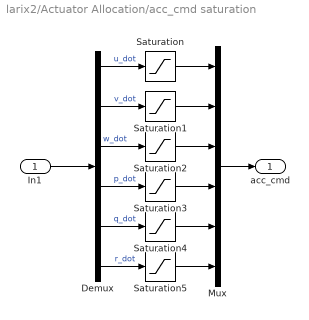
== system larix2/Actuator Allocation/acc_cmd saturation ==
  In1 : Inport
  Demux : Demux  Outputs=6
  Mux : Mux  Inputs=6
  Saturation : Saturate  UpperLimit=blimp.prp.du_max  LowerLimit=-blimp.prp.du_max
  Saturation1 : Saturate  UpperLimit=blimp.prp.dv_max  LowerLimit=-blimp.prp.dv_max
  Saturation2 : Saturate  UpperLimit=blimp.prp.dw_max  LowerLimit=-blimp.prp.dw_max
  Saturation3 : Saturate  UpperLimit=blimp.prp.dp_max  LowerLimit=-blimp.prp.dp_max
  Saturation4 : Saturate  UpperLimit=blimp.prp.dq_max  LowerLimit=-blimp.prp.dq_max
  Saturation5 : Saturate  UpperLimit=blimp.prp.dr_max  LowerLimit=-blimp.prp.dr_max
  acc_cmd : Outport
  wires:
  In1/1 -> Demux/1
  Mux/1 -> acc_cmd/1
  Demux/1 -> Saturation/1  "u_dot"
  Saturation/1 -> Mux/1
  Demux/2 -> Saturation1/1  "v_dot"
  Saturation1/1 -> Mux/2
  Demux/3 -> Saturation2/1  "w_dot"
  Saturation2/1 -> Mux/3
  Demux/4 -> Saturation3/1  "p_dot"
  Saturation3/1 -> Mux/4
  Demux/5 -> Saturation4/1  "q_dot"
  Saturation4/1 -> Mux/5
  Demux/6 -> Saturation5/1  "r_dot"
  Saturation5/1 -> Mux/6

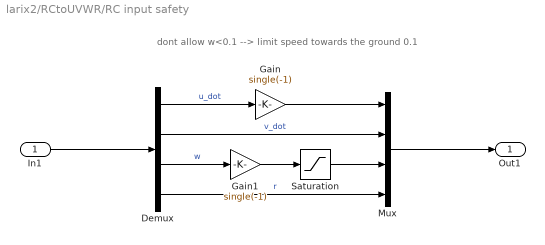
== system larix2/RCtoUVWR/RC input safety ==
  note: dont allow w<0.1 --> limit speed towards the ground
      |
      |  0.1
  In1 : Inport
  Demux : Demux
  Gain : Gain  Gain=single(-1)
  Gain1 : Gain  Gain=single(-1)
  Mux : Mux
  Saturation : Saturate  UpperLimit=0.2  LowerLimit=-1
  Out1 : Outport
  wires:
  In1/1 -> Demux/1
  Mux/1 -> Out1/1
  Demux/1 -> Gain/1  "u_dot"
  Demux/2 -> Mux/2  "v_dot"
  Demux/4 -> Mux/4  "r"
  Demux/3 -> Gain1/1  "w"
  Saturation/1 -> Mux/3
  Gain/1 -> Mux/1
  Gain1/1 -> Saturation/1

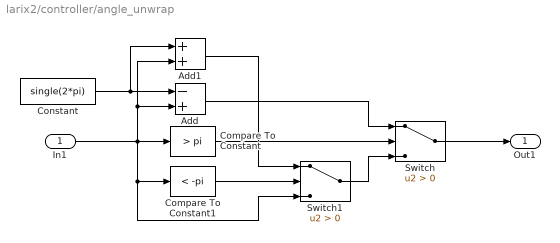
== system larix2/controller/angle_unwrap ==
  In1 : Inport
  Add : Sum  Inputs=-+
  Add1 : Sum
  Compare To Constant : simulink/Logic and Bit Operations/Compare To Constant  relop=>  const=pi  OutDataTypeStr=boolean
  Compare To Constant1 : simulink/Logic and Bit Operations/Compare To Constant  relop=<  const=-pi  OutDataTypeStr=boolean
  Constant : Constant  Value=single(2*pi)
  Switch : Switch  Criteria=u2 > Threshold
  Switch1 : Switch  Criteria=u2 > Threshold
  Out1 : Outport
  wires:
  In1/1 -> Switch1/3, Compare To Constant1/1, Compare To Constant/1, Add1/2, Add/2
  Compare To Constant/1 -> Switch/2
  Constant/1 -> Add/1, Add1/1
  Add/1 -> Switch/1
  Compare To Constant1/1 -> Switch1/2
  Switch/1 -> Out1/1
  Switch1/1 -> Switch/3
  Add1/1 -> Switch1/1

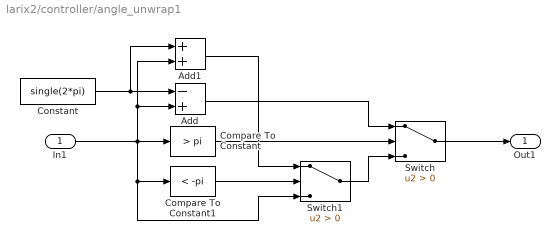
== system larix2/controller/angle_unwrap1 ==
  In1 : Inport
  Add : Sum  Inputs=-+
  Add1 : Sum
  Compare To Constant : simulink/Logic and Bit Operations/Compare To Constant  relop=>  const=pi  OutDataTypeStr=boolean
  Compare To Constant1 : simulink/Logic and Bit Operations/Compare To Constant  relop=<  const=-pi  OutDataTypeStr=boolean
  Constant : Constant  Value=single(2*pi)
  Switch : Switch  Criteria=u2 > Threshold
  Switch1 : Switch  Criteria=u2 > Threshold
  Out1 : Outport
  wires:
  In1/1 -> Switch1/3, Compare To Constant1/1, Compare To Constant/1, Add1/2, Add/2
  Compare To Constant/1 -> Switch/2
  Constant/1 -> Add/1, Add1/1
  Add/1 -> Switch/1
  Compare To Constant1/1 -> Switch1/2
  Switch/1 -> Out1/1
  Switch1/1 -> Switch/3
  Add1/1 -> Switch1/1

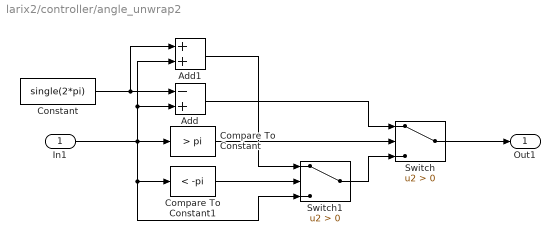
== system larix2/controller/angle_unwrap2 ==
  In1 : Inport
  Add : Sum  Inputs=-+
  Add1 : Sum
  Compare To Constant : simulink/Logic and Bit Operations/Compare To Constant  relop=>  const=pi  OutDataTypeStr=boolean
  Compare To Constant1 : simulink/Logic and Bit Operations/Compare To Constant  relop=<  const=-pi  OutDataTypeStr=boolean
  Constant : Constant  Value=single(2*pi)
  Switch : Switch  Criteria=u2 > Threshold
  Switch1 : Switch  Criteria=u2 > Threshold
  Out1 : Outport
  wires:
  In1/1 -> Switch1/3, Compare To Constant1/1, Compare To Constant/1, Add1/2, Add/2
  Compare To Constant/1 -> Switch/2
  Constant/1 -> Add/1, Add1/1
  Add/1 -> Switch/1
  Compare To Constant1/1 -> Switch1/2
  Switch/1 -> Out1/1
  Switch1/1 -> Switch/3
  Add1/1 -> Switch1/1

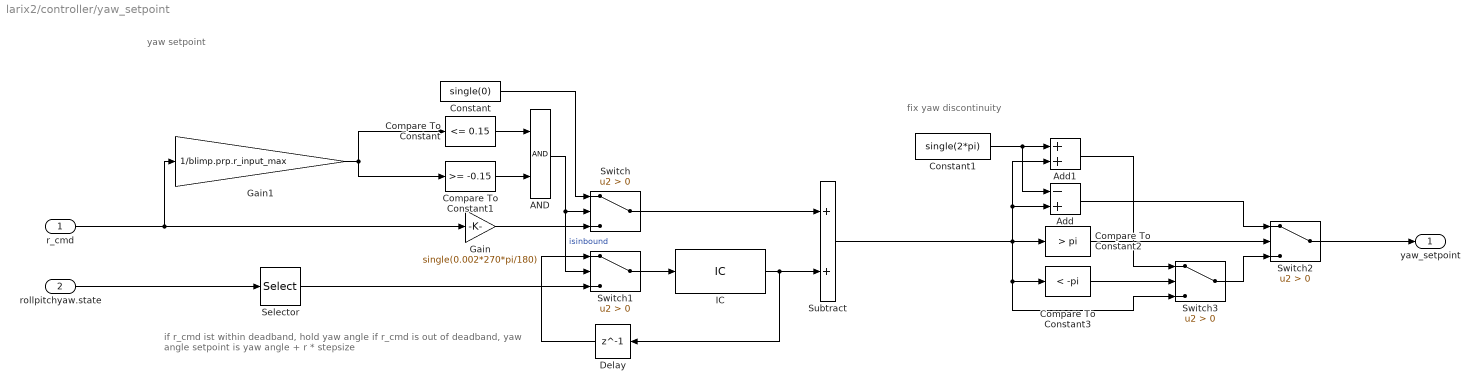
== system larix2/controller/yaw_setpoint ==
  note: fix yaw discontinuity
  note: yaw setpoint
  note: if r_cmd ist within deadband, hold yaw angle
      | if r_cmd is out of deadband, yaw angle setpoint is yaw angle + r * stepsize
  r_cmd : Inport
  rollpitchyaw.state : Inport  Port=2
  AND : Logic  AllPortsSameDT=off  OutDataTypeStr=boolean
  Add : Sum  Inputs=-+
  Add1 : Sum
  Compare To Constant : simulink/Logic and Bit Operations/Compare To Constant  relop=<=  const=0.15  OutDataTypeStr=boolean
  Compare To Constant1 : simulink/Logic and Bit Operations/Compare To Constant  relop=>=  const=-0.15  OutDataTypeStr=boolean
  Compare To Constant2 : simulink/Logic and Bit Operations/Compare To Constant  relop=>  const=pi  OutDataTypeStr=boolean
  Compare To Constant3 : simulink/Logic and Bit Operations/Compare To Constant  relop=<  const=-pi  OutDataTypeStr=boolean
  Constant : Constant  Value=single(0)
  Constant1 : Constant  Value=single(2*pi)
  Delay : Delay  DelayLength=1
  Gain : Gain  Gain=single(0.002*270*pi/180)
  Gain1 : Gain  Gain=1/blimp.prp.r_input_max
  IC : InitialCondition  Value=single(eul_0(3))
  Selector : Selector  InputPortWidth=3  IndexOptions=Index vector (dialog)  Indices=[3]  OutputSizes=1
  Subtract : Sum
  Switch{,1..3} (4 alike) : Switch  Criteria=u2 > Threshold
  yaw_setpoint : Outport
  wires:
  r_cmd/1 -> Gain1/1, Gain/1
  Compare To Constant/1 -> AND/1
  Compare To Constant1/1 -> AND/2
  AND/1 -> Switch/2, Switch1/2  "isinbound"
  Constant/1 -> Switch/1
  Switch/1 -> Subtract/1
  rollpitchyaw.state/1 -> Selector/1
  Selector/1 -> Switch1/3
  Switch1/1 -> IC/1
  Gain/1 -> Switch/3
  Gain1/1 -> Compare To Constant/1, Compare To Constant1/1
  Delay/1 -> Switch1/1
  IC/1 -> Delay/1, Subtract/2
  Subtract/1 -> Switch3/3, Compare To Constant3/1, Add1/2, Add/2, Compare To Constant2/1
  Add1/1 -> Switch3/1
  Compare To Constant3/1 -> Switch3/2
  Constant1/1 -> Add/1, Add1/1
  Switch2/1 -> yaw_setpoint/1
  Add/1 -> Switch2/1
  Compare To Constant2/1 -> Switch2/2
  Switch3/1 -> Switch2/3

== matlab function larix2/Actuator Allocation/acc_allocation ==
  data: euler input; acc_cmd input; F output size=4; blimp parameter
function F = fcn(euler, acc_cmd, blimp)

% accellerations in BFG cs
u_dot = acc_cmd(1);
%v_dot = acc_cmd(2);
w_dot = acc_cmd(3);
p_dot = acc_cmd(4);  
%q_dot = acc_cmd(5);
r_dot = acc_cmd(6);

roll = euler(1);
pitch = euler(2);


%ALLOCATION
                            % [-1 1]        stick accounts for pitch movement -> stays level
if w_dot <= 0
    Thrustvector_angle = atan2(-(w_dot/cos(roll)),u_dot)*2/pi -1;  %neg towards front
else
    Thrustvector_angle = atan2(-(w_dot/cos(roll)),u_dot)*2/pi +1;
end

stick = Thrustvector_angle - pitch*2/pi;

%TF_BFtoBFG = eul2rotm([roll pitch 0],'XYZ')';   

%normalized accelerations
u_dot_norm = u_dot;
w_dot_norm = w_dot/cos(roll);

p_dot_norm = p_dot/(cos(Thrustvector_angle)*blimp.prp.length_stick);
r_dot_norm = r_dot/(cos(roll)*(abs(blimp.par.bot_rud_motor.position(1))));

acc_norm = single([u_dot_norm, 0, w_dot_norm, p_dot_norm, 0, r_dot_norm]);
acc_norm(isnan(acc_norm)) = 0;

%inertia_ax_bfg = TF_BFtoBFG * blimp.mM.M(1:3,1:3) * TF_BFtoBFG';        %transform axial and rotational inertia into BFG coordinates
%inertia_rot_bfg = TF_BFtoBFG * blimp.mM.M(4:6,4:6) * TF_BFtoBFG';
inertia_ax_bfg = blimp.mM.M(1:3,1:3);        %transform axial and rotational inertia into BFG coordinates
inertia_rot_bfg = blimp.mM.M(4:6,4:6);


%multiply by mass matrix to get actual needed force
FT_norm = acc_norm.*[diag(inertia_ax_bfg); diag(inertia_rot_bfg)]';

FLRuw = sign(FT_norm(3))*sqrt(FT_norm(1)^2 + FT_norm(3)^2);
FLRp = FT_norm(4);
F3r = FT_norm(6);

F3 = F3r;
%F3= -0.18;
%F3= 0.7

%enforce saturation safety bounds


%if F3 comes too close to saturation, decrease delta FLR
%works for "u minmal v movement" and "u allowed v movement"
if (F3 < blimp.prp.FB_min*blimp.prp.FB_softboundmargin) && (blimp.prp.FB_min < F3) &&(FLRp > 0)
    delta_bound = (blimp.prp.FB_min - F3)/((1-blimp.prp.FB_softboundmargin)*blimp.prp.FB_min); % = distance from hard bound / distance from hard bound at the beginning of th safetymargin 
elseif (F3 > blimp.prp.FB_max*blimp.prp.FB_softboundmargin) && (blimp.prp.FB_max > F3)&& (FLRp < 0)
    delta_bound = (blimp.prp.FB_max - F3)/((1-blimp.prp.FB_softboundmargin)*blimp.prp.FB_max);
elseif (blimp.prp.FB_min > F3) && (FLRp > 0)
    F3 = blimp.prp.FB_min;
    delta_bound = single(0);
elseif (blimp.prp.FB_max < F3) && (FLRp < 0)
    F3 = blimp.prp.FB_max;
    delta_bound = single(0);
else
    delta_bound = single(1);
end
    FLRp = FLRp*(1-0.6*(1-delta_bound)^2);
    
    

if (FLRuw/2 + abs(FLRp/2)) > blimp.prp.FL_max*blimp.prp.FLR_safetymargin          %include case if maximum is passed?
    if FLRp > 0
        FRp = blimp.prp.FR_max*blimp.prp.FLR_safetymargin;          % set trust to the minimal possible value on the side where the blimp should move to
        FLp = -FLRp + blimp.prp.FR_max*blimp.prp.FLR_safetymargin;       %calculate trust on the left side so that the resulting torque still comes out to the desired value even tho the thrust on the other side has hit the bound
        if (FLp + FRp) < FLRuw                                              %make sure the offset between FL and FR is never greater than the desired up/forward force since that would mean drift
            FLp = FLRuw - blimp.prp.FR_max*blimp.prp.FLR_safetymargin;
        end
        if FLp < blimp.prp.FL_min*blimp.prp.FLR_safetymargin            
            FLp = blimp.prp.FL_min*blimp.prp.FLR_safetymargin;          %hard limit  --> doesnt mean control is lost
        end
    else       
        FLp = blimp.prp.FR_max*blimp.prp.FLR_safetymargin; 
        FRp = FLRp + blimp.prp.FL_max*blimp.prp.FLR_safetymargin;      % the same thing as before but for the other movement direction
        if (FLp + FRp) < FLRuw                                             
            FRp = FLRuw - blimp.prp.FR_max*blimp.prp.FLR_safetymargin;
        end
        if FRp < blimp.prp.FR_min*blimp.prp.FLR_safetymargin
            FRp = blimp.prp.FR_min*blimp.prp.FLR_safetymargin;
        end
    end
    FLRuw = FLRuw - (FLp + FRp);                                        %subtract the difference of left and right thrust from the uw thrust to ensure correct trust (no w drift)
else
    FLp = -FLRp/2;
    FRp = FLRp/2;
end

FL = FLRuw/2 + FLp; 
FR = FLRuw/2 + FRp; 


LRS3 = [FL FR stick F3];

F = LRS3(1,:)'
